simulink model "hexAeroCoefficientsModelTestHarness"  (R2024a)
settings: configuration reference "standardSILConfiguraitonParams" (kept outside this file)
settings Model: Creator=GTAR  LastModifiedBy=jerem
settings ConfigSetRef: SourceName=standardSILConfiguraitonParams  SourceLocation=Base Workspace

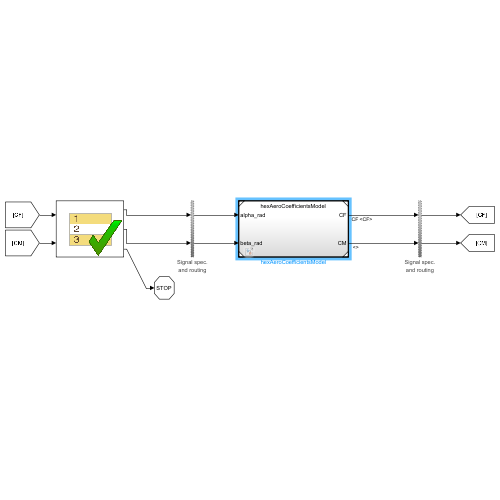
[thumbnail: Simulink's stored preview of the top-level diagram]
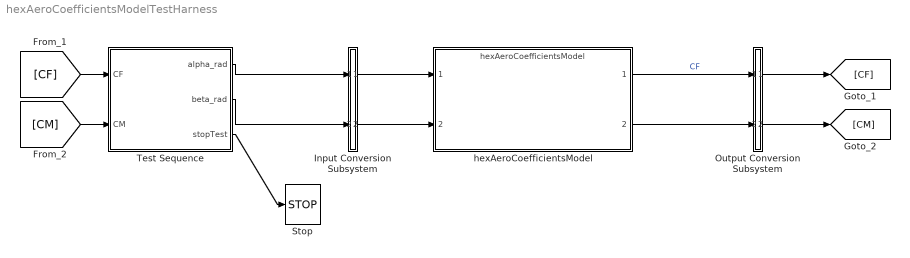
== system hexAeroCoefficientsModelTestHarness ==
  Input Conversion Subsystem : Subsystem  Tag=__SLT_ICS__  Description=|
      | Signal spec.
      | and routing
      settings: AttributesFormatString=%<Description>
  Output Conversion Subsystem : Subsystem  Tag=__SLT_OCS__  Description=|
      | Signal spec.
      | and routing
      settings: AttributesFormatString=%<Description>
  Stop : Stop
  Test Sequence : Test Sequence  TreatAsAtomicUnit=on
  hexAeroCoefficientsModel : ModelReference  ModelNameDialog=hexAeroCoefficientsModel  SimulationMode=Normal  ModelReferenceVersion=1.11
  wires:
  Test Sequence/1(alpha_rad) -> Input Conversion Subsystem/1(Inport_1)
  Test Sequence/2(beta_rad) -> Input Conversion Subsystem/2(Inport_2)
  [CF] -> Test Sequence/1(CF)
  [CM] -> Test Sequence/2(CM)
  Output Conversion Subsystem/1(Outport_1) -> [CF]
  Output Conversion Subsystem/2(Outport_2) -> [CM]
  Input Conversion Subsystem/1(Outport_1) -> hexAeroCoefficientsModel/1
  Input Conversion Subsystem/2(Outport_2) -> hexAeroCoefficientsModel/2
  hexAeroCoefficientsModel/1 -> Output Conversion Subsystem/1(Inport_1)  "CF"
  hexAeroCoefficientsModel/2 -> Output Conversion Subsystem/2(Inport_2)
  Test Sequence/3(stopTest) -> Stop/1

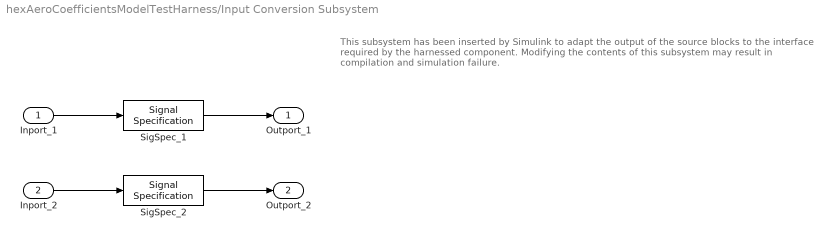
== system hexAeroCoefficientsModelTestHarness/Input Conversion Subsystem ==
  note: This subsystem has been inserted by Simulink to adapt the output of the source blocks to the interface required by the harnessed component.
      |  Modifying the contents of this subsystem may result in compilation and simulation failure.
  Inport_1 : Inport
  Inport_2 : Inport  Port=2
  SigSpec_1 : SignalSpecification  OutDataTypeStr=double  Dimensions=[1]  SampleTime=[-1, 0]
  SigSpec_2 : SignalSpecification  OutDataTypeStr=double  Dimensions=[1]  SampleTime=[-1, 0]
  Outport_1 : Outport
  Outport_2 : Outport  Port=2
  wires:
  SigSpec_1/1 -> Outport_1/1
  Inport_1/1 -> SigSpec_1/1
  SigSpec_2/1 -> Outport_2/1
  Inport_2/1 -> SigSpec_2/1

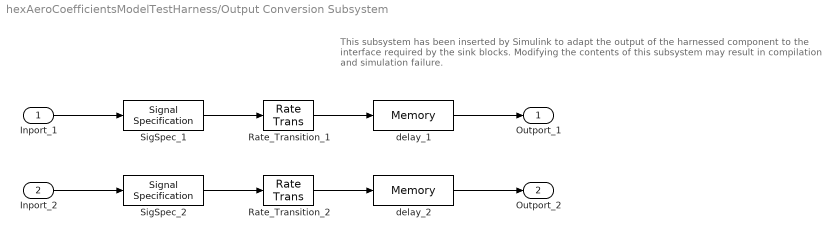
== system hexAeroCoefficientsModelTestHarness/Output Conversion Subsystem ==
  note: This subsystem has been inserted by Simulink to adapt the output of the harnessed component to the interface required by the sink blocks.
      |  Modifying the contents of this subsystem may result in compilation and simulation failure.
  Inport_1 : Inport
  Inport_2 : Inport  Port=2
  Rate_Transition_1 : RateTransition  OutPortSampleTimeOpt=Inherit
  Rate_Transition_2 : RateTransition  OutPortSampleTimeOpt=Inherit
  SigSpec_1 : SignalSpecification  OutDataTypeStr=double  Dimensions=[3]
  SigSpec_2 : SignalSpecification  OutDataTypeStr=double  Dimensions=[3]
  delay_1 : Memory
  delay_2 : Memory
  Outport_1 : Outport
  Outport_2 : Outport  Port=2
  wires:
  Inport_1/1 -> SigSpec_1/1
  SigSpec_1/1 -> Rate_Transition_1/1
  Rate_Transition_1/1 -> delay_1/1
  delay_1/1 -> Outport_1/1
  Inport_2/1 -> SigSpec_2/1
  SigSpec_2/1 -> Rate_Transition_2/1
  Rate_Transition_2/1 -> delay_2/1
  delay_2/1 -> Outport_2/1

== stateflow chart hexAeroCoefficientsModelTestHarness/Test Sequence ==
  state Scenario_1
    state Initialize
      %% Initialize data outputs.
      alpha_rad = 0;
      beta_rad = 0;
      stopTest = false;
    state setNoseDn
      alpha_rad = -0.1;
      beta_rad = 0;
    state checkNoseDn
      %CX -
      %CY 0
      %CZ +
      verify(CF(1) < 0)
      verify(isClose(CF(2), 0))
      verify(CF(3) > 0)
      verify(isClose(CM(1), 0))
      verify(isClose(CM(2), 0))
      verify(isClose(CM(3), 0))
    state setNoseUp
      alpha_rad = 0.1;
      beta_rad = 0;
    state checkNoseUp
      %CX -
      %CY 0
      %CZ -
      verify(CF(1) < 0)
      verify(isClose(CF(2), 0))
      verify(CF(3) < 0)
      verify(isClose(CM(1), 0))
      verify(isClose(CM(2), 0))
      verify(isClose(CM(3), 0))
    state setNoseDnLeft
      alpha_rad = -0.1;
      beta_rad = 0.1;
    state checkNoseDnLeft
      %CX -
      %CY -
      %CZ +
      verify(CF(1) < 0)
      verify(CF(2) < 0)
      verify(CF(3) > 0)
      verify(isClose(CM(1), 0))
      verify(isClose(CM(2), 0))
      verify(isClose(CM(3), 0))
    state setNoseDnRight
      alpha_rad = -0.1;
      beta_rad = -0.1;
    state checkNoseDnRight
      %CX -
      %CY +
      %CZ +
      verify(CF(1) < 0)
      verify(CF(2) > 0)
      verify(CF(3) > 0)
      verify(isClose(CM(1), 0))
      verify(isClose(CM(2), 0))
      verify(isClose(CM(3), 0))
    state EndTest
      stopTest = true;
    (default) -> Initialize
    Initialize -> setNoseDn : [
        | true
        | ]
    setNoseDn -> checkNoseDn : [
        | after(1, sec)
        | ]
    checkNoseDn -> setNoseUp : [
        | true
        | ]
    setNoseUp -> checkNoseUp : [
        | after(1, sec)
        | ]
    checkNoseUp -> setNoseDnLeft : [
        | true
        | ]
    setNoseDnLeft -> checkNoseDnLeft : [
        | after(1, sec)
        | ]
    checkNoseDnLeft -> setNoseDnRight : [
        | true
        | ]
    setNoseDnRight -> checkNoseDnRight : [
        | after(1, sec)
        | ]
    checkNoseDnRight -> EndTest : [
        | true
        | ]
  (default) -> Scenario_1 : {assert(Active_Scenario_Index == 1,'The value of Scenario Parameter ''Active_Scenario_Index'' is not valid. Use the index of the scenario to specify it.')}
  data: CF input double size=[3]; CM input double size=[3]; alpha_rad output double size=[1]; beta_rad output double size=[1]; stopTest output; Active_Scenario_Index parameter =1
